simulink model "PANCL"  (R2020a)
settings: Solver=ode45  StartTime=0.0  StopTime=10.0  RelTol=1e-3  EnableMultiTasking=on
settings Model: Creator=CARVALHO  LastModifiedBy=Arnaldo
settings DataIOCC: LimitDataPoints=on  SaveFormat=Array  ReturnWorkspaceOutputs=off
settings OptimizationCC: LifeSpan=inf
settings DebuggingCC: SFUnexpectedBacktrackingDiag=warning  SFNoUnconditionalDefaultTransitionDiag=warning  SFExecutionAtInitializationDiag=none  ArithmeticOperatorsInVariantConditions=warning
settings HardwareCC: ProdBitPerPointer=32  ProdBitPerSizeT=32  ProdBitPerPtrDiffT=32  ProdLargestAtomicFloat=None  ProdIntDivRoundTo=Undefined  ProdEndianess=Unspecified  ProdWordSize=32  ProdHWDeviceType=32-bit Generic
settings ModelReferenceCC: PropagateSignalLabelsOutOfModel=off
settings SFSimCC: SimUseLocalCustomCode=off  CustomCodeUndefinedFunction=UseInterfaceOnly
settings RTWCC: RTWUseLocalCustomCode=off
settings CodeAppCC: StateflowObjectComments=on
settings GRTTargetCC: TargetLangStandard=C89/C90 (ANSI)
settings ConfigComp: CovMetricSettings=dw  CovHtmlReporting=on  CovSaveCumulativeToWorkspaceVar=on  CovSaveSingleToWorkspaceVar=on  CovExternalEMLEnable=off

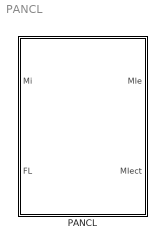
== system PANCL ==
  PANCL : Subsystem  Tag=NAP  Description=Célula de Aprendizagem NAP

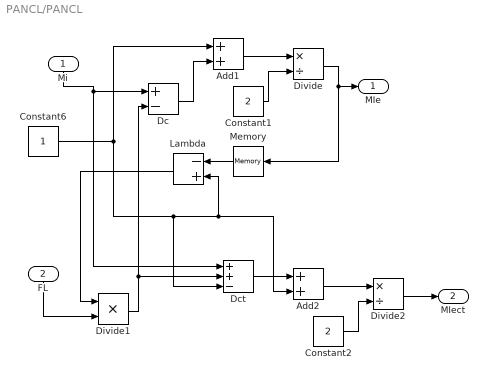
== system PANCL/PANCL ==
  Mi : Inport
  FL : Inport  Port=2
  Add1 : Sum
  Add2 : Sum
  Constant1 : Constant  Value=2
  Constant2 : Constant  Value=2
  Constant6 : Constant
  Dc : Sum  Inputs=+-
  Dct : Sum  Inputs=++-
  Divide : Product  Inputs=*/
  Divide1 : Product  Inputs=**
  Divide2 : Product  Inputs=*/
  Lambda : Sum  Inputs=-+
  Memory : Memory  LinearizeAsDelay=on
  MIe : Outport
  MIect : Outport  Port=2
  wires:
  Dc/1 -> Add1/2
  Add1/1 -> Divide/1
  Constant1/1 -> Divide/2
  Divide/1 -> Memory/1, MIe/1
  Memory/1 -> Lambda/1
  Constant6/1 -> Add2/2, Lambda/2, Dct/3, Add1/1
  Mi/1 -> Dc/1, Dct/1
  Divide1/1 -> Dct/2, Dc/2
  FL/1 -> Divide1/2
  Lambda/1 -> Divide1/1
  Dct/1 -> Add2/1
  Add2/1 -> Divide2/1
  Constant2/1 -> Divide2/2
  Divide2/1 -> MIect/1
